simulink model "ModernControlSimOpenLoop"  (R2013a)
settings: Solver=ode4  StartTime=Tstart  StopTime=Tfinal  FixedStep=Ts  RelTol=1e-3
values from neighbouring files (symbols this model uses):
  A = [0  1  0  0 ... (first row only)    [ModernControlSim.m]
  B = [0 ... (first row only)    [ModernControlSim.m]
  N_bar = (b1*K(3)-a2)/b1    [ModernControlSim.m]
undefined symbols (not defined in the file or in its folder): K_temp
settings Model: BufferReuse=off  Creator=ML-07  LastModifiedBy=econ
settings DataIOCC: SignalLoggingSaveFormat=ModelDataLogs
settings OptimizationCC: InlineParams=on  BufferReuse=off  ExpressionDepthLimit=2147483647
settings DebuggingCC: MultiTaskDSMMsg=warning  MultiTaskCondExecSysMsg=none  FcnCallInpInsideContextMsg=EnableAllAsWarning  InitInArrayFormatMsg=none  StrictBusMsg=None
settings RTWCC: IncludeERTFirstTime=on
settings GRTTargetCC: CodeReplacementLibrary=None  CombineOutputUpdateFcns=off  CPPClassGenCompliant=on  GRTInterface=on

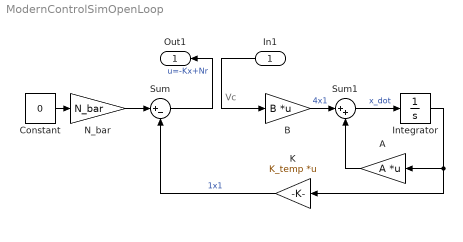
== system ModernControlSimOpenLoop ==
  note: Vc
  In1 : Inport
  A : Gain  Gain=A  Multiplication=Matrix(K*u)
  B : Gain  Gain=B  Multiplication=Matrix(K*u)
  Constant : Constant  Value=0
  Integrator : Integrator  InitialCondition=0.00000000001
  K : Gain  Gain=K_temp  Multiplication=Matrix(K*u)
  N_bar : Gain  Gain=N_bar
  Sum : Sum  Inputs=|+-
  Sum1 : Sum  Inputs=|++
  Out1 : Outport
  wires:
  Sum1/1 -> Integrator/1  "x_dot"
  Integrator/1 -> K/1, A/1
  A/1 -> Sum1/2
  B/1 -> Sum1/1  "4x1"
  K/1 -> Sum/2  "1x1"
  Constant/1 -> N_bar/1
  N_bar/1 -> Sum/1
  In1/1 -> B/1
  Sum/1 -> Out1/1  "u=-Kx+Nr"
